simulink model "test_integration_decrease_power"  (R2022b)
settings: Solver=FixedStepAuto  StartTime=0.0  StopTime=240  FixedStep=0.1  RelTol=1e-3
settings Model: Creator=cristian  LastModifiedBy=cristian
settings ConfigComp: CovScope=ReferencedModels  CovIncludeTopModel=off  CovHTMLOptions=-sRT=1 -sVT=0 -aTS=1 -agT=1 -bRG=1 -bTC=1 -hTR=0 -nFC=0 -nFD=1 -scm=1 -bcm=1 -xEv=0 -xEM=0 -req=1  CovEnableCumulative=off

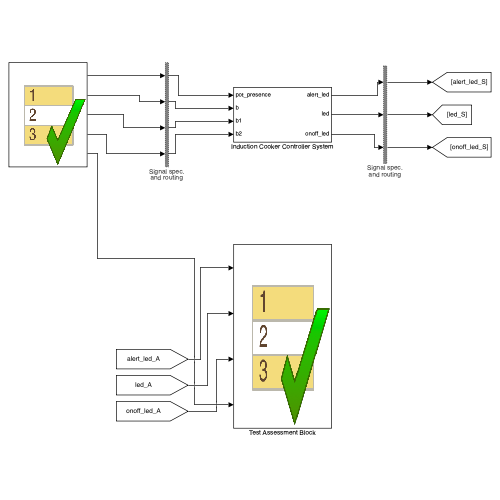
[thumbnail: Simulink's stored preview of the top-level diagram]
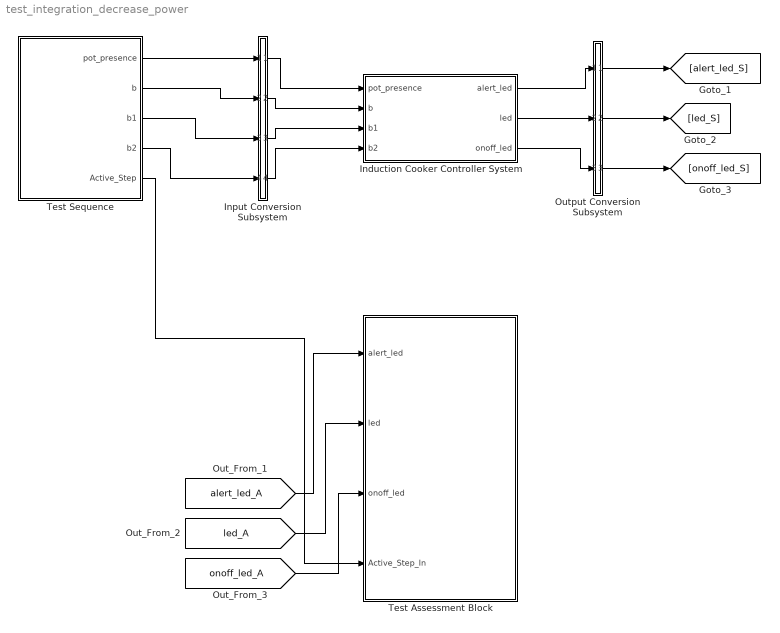
== system test_integration_decrease_power ==
  Induction Cooker Controller System : Subsystem
  Input Conversion Subsystem : Subsystem  Tag=__SLT_ICS__  Description=|
      | Signal spec.
      | and routing
      settings: AttributesFormatString=%<Description>
  Output Conversion Subsystem : Subsystem  Tag=__SLT_OCS__  Description=|
      | Signal spec.
      | and routing
      settings: AttributesFormatString=%<Description>
  Test Assessment Block : Test Sequence  Tag=__SLT_ASMT__  TreatAsAtomicUnit=on
  Test Sequence : Test Sequence  TreatAsAtomicUnit=on
  wires:
  [alert_led_A] -> Test Assessment Block/1(alert_led)
  [led_A] -> Test Assessment Block/2(led)
  [onoff_led_A] -> Test Assessment Block/3(onoff_led)
  Test Sequence/1(pot_presence) -> Input Conversion Subsystem/1(Inport_1)
  Test Sequence/2(b) -> Input Conversion Subsystem/2(Inport_2)
  Test Sequence/3(b1) -> Input Conversion Subsystem/3(Inport_3)
  Test Sequence/4(b2) -> Input Conversion Subsystem/4(Inport_4)
  Output Conversion Subsystem/1(Outport_1) -> [alert_led_S]
  Output Conversion Subsystem/2(Outport_2) -> [led_S]
  Output Conversion Subsystem/3(Outport_3) -> [onoff_led_S]
  Input Conversion Subsystem/1(Outport_1) -> Induction Cooker Controller System/1(pot_presence)
  Input Conversion Subsystem/2(Outport_2) -> Induction Cooker Controller System/2(b)
  Input Conversion Subsystem/3(Outport_3) -> Induction Cooker Controller System/3(b1)
  Input Conversion Subsystem/4(Outport_4) -> Induction Cooker Controller System/4(b2)
  Induction Cooker Controller System/1(alert_led) -> Output Conversion Subsystem/1(Inport_1)
  Induction Cooker Controller System/2(led) -> Output Conversion Subsystem/2(Inport_2)
  Induction Cooker Controller System/3(onoff_led) -> Output Conversion Subsystem/3(Inport_3)
  Test Sequence/5(Active_Step) -> Test Assessment Block/4(Active_Step_In)

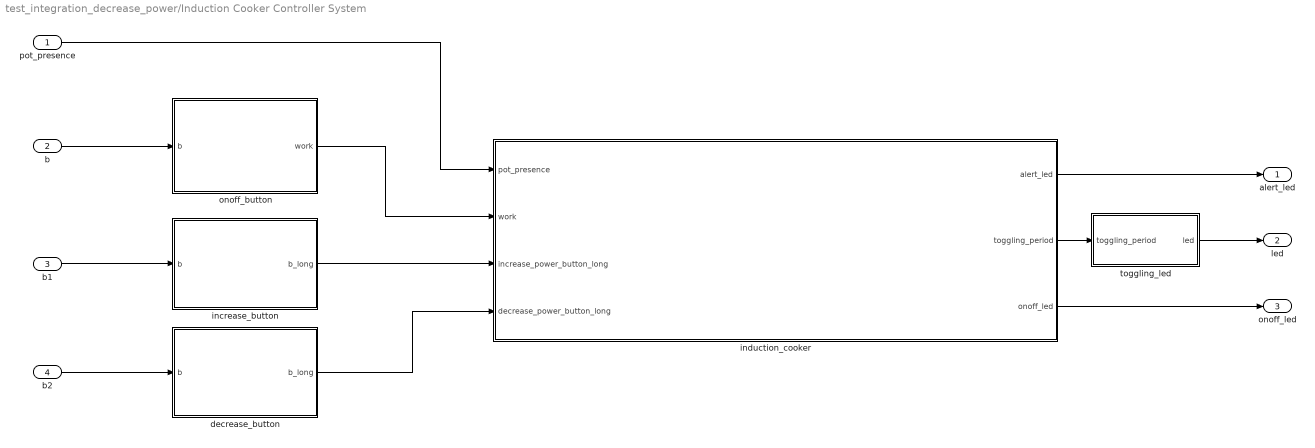
== system test_integration_decrease_power/Induction Cooker Controller System ==
  pot_presence : Inport
  b : Inport  Port=2
  b1 : Inport  Port=3
  b2 : Inport  Port=4
  decrease_button : Stateflow chart  TreatAsAtomicUnit=on
  increase_button : Stateflow chart  TreatAsAtomicUnit=on
  induction_cooker : Stateflow chart  TreatAsAtomicUnit=on
  onoff_button : Stateflow chart  TreatAsAtomicUnit=on
  toggling_led : Stateflow chart  TreatAsAtomicUnit=on
  alert_led : Outport
  led : Outport  Port=2
  onoff_led : Outport  Port=3
  wires:
  decrease_button/1(b_long) -> induction_cooker/4(decrease_power_button_long)
  increase_button/1(b_long) -> induction_cooker/3(increase_power_button_long)
  induction_cooker/2(toggling_period) -> toggling_led/1(toggling_period)
  toggling_led/1(led) -> led/1
  b1/1 -> increase_button/1(b)
  induction_cooker/3(onoff_led) -> onoff_led/1
  onoff_button/1(work) -> induction_cooker/2(work)
  b2/1 -> decrease_button/1(b)
  induction_cooker/1(alert_led) -> alert_led/1
  pot_presence/1 -> induction_cooker/1(pot_presence)
  b/1 -> onoff_button/1(b)

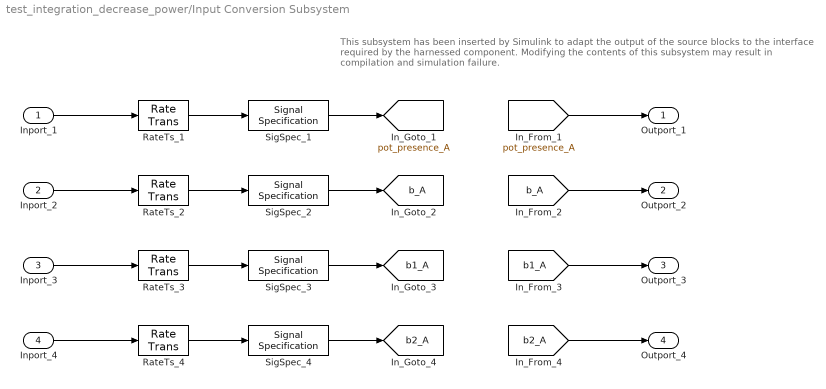
== system test_integration_decrease_power/Input Conversion Subsystem ==
  note: This subsystem has been inserted by Simulink to adapt the output of the source blocks to the interface required by the harnessed component.
      |  Modifying the contents of this subsystem may result in compilation and simulation failure.
  Inport_1 : Inport
  Inport_2 : Inport  Port=2
  Inport_3 : Inport  Port=3
  Inport_4 : Inport  Port=4
  RateTs_{1..4} (4 alike) : RateTransition  OutPortSampleTime=[-1, 0]
  SigSpec_{1..4} (4 alike) : SignalSpecification  OutDataTypeStr=boolean  Dimensions=[1]  SampleTime=[-1, 0]
  Outport_1 : Outport
  Outport_2 : Outport  Port=2
  Outport_3 : Outport  Port=3
  Outport_4 : Outport  Port=4
  tag scope: b1_A=global, b2_A=global, b_A=global, pot_presence_A=global
  wires:
  [pot_presence_A] -> Outport_1/1
  SigSpec_1/1 -> [pot_presence_A]
  RateTs_1/1 -> SigSpec_1/1
  Inport_1/1 -> RateTs_1/1
  [b_A] -> Outport_2/1
  SigSpec_2/1 -> [b_A]
  RateTs_2/1 -> SigSpec_2/1
  Inport_2/1 -> RateTs_2/1
  [b1_A] -> Outport_3/1
  SigSpec_3/1 -> [b1_A]
  RateTs_3/1 -> SigSpec_3/1
  Inport_3/1 -> RateTs_3/1
  [b2_A] -> Outport_4/1
  SigSpec_4/1 -> [b2_A]
  RateTs_4/1 -> SigSpec_4/1
  Inport_4/1 -> RateTs_4/1

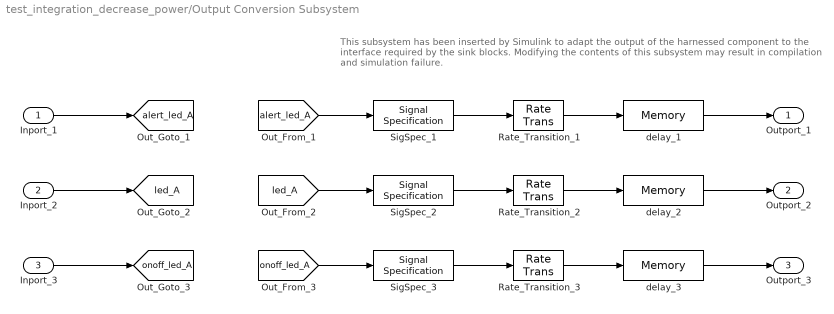
== system test_integration_decrease_power/Output Conversion Subsystem ==
  note: This subsystem has been inserted by Simulink to adapt the output of the harnessed component to the interface required by the sink blocks.
      |  Modifying the contents of this subsystem may result in compilation and simulation failure.
  Inport_1 : Inport
  Inport_2 : Inport  Port=2
  Inport_3 : Inport  Port=3
  Rate_Transition_1 : RateTransition  OutPortSampleTimeOpt=Inherit
  Rate_Transition_2 : RateTransition  OutPortSampleTimeOpt=Inherit
  Rate_Transition_3 : RateTransition  OutPortSampleTimeOpt=Inherit
  SigSpec_1 : SignalSpecification  OutDataTypeStr=boolean  Dimensions=[1]
  SigSpec_2 : SignalSpecification  OutDataTypeStr=boolean  Dimensions=[1]
  SigSpec_3 : SignalSpecification  OutDataTypeStr=boolean  Dimensions=[1]
  delay_1 : Memory
  delay_2 : Memory
  delay_3 : Memory
  Outport_1 : Outport
  Outport_2 : Outport  Port=2
  Outport_3 : Outport  Port=3
  tag scope: alert_led_A=global, led_A=global, onoff_led_A=global
  wires:
  Inport_1/1 -> [alert_led_A]
  [alert_led_A] -> SigSpec_1/1
  SigSpec_1/1 -> Rate_Transition_1/1
  Rate_Transition_1/1 -> delay_1/1
  delay_1/1 -> Outport_1/1
  Inport_2/1 -> [led_A]
  [led_A] -> SigSpec_2/1
  SigSpec_2/1 -> Rate_Transition_2/1
  Rate_Transition_2/1 -> delay_2/1
  delay_2/1 -> Outport_2/1
  Inport_3/1 -> [onoff_led_A]
  [onoff_led_A] -> SigSpec_3/1
  SigSpec_3/1 -> Rate_Transition_3/1
  Rate_Transition_3/1 -> delay_3/1
  delay_3/1 -> Outport_3/1

== stateflow chart test_integration_decrease_power/Induction Cooker Controller System/decrease_button ==
  note: Bottone a livelli, la pressione per un numero di secondi pari a DURATION permette di avere un uscita alta in maniera istantanea.
      | Per avere in output un valore PRESSED, è necessare lasciare il bottone e premere tra un output e l'altro.
  state Wait
    en: b_long = RELEASED
  state Pressed
    en: b_long = RELEASED;
    on after(DURATION,sec): b_long = PRESSED
  state LongPressed
    en: b_long = RELEASED
  (default) -> Wait
  Wait -> Pressed : [b == PRESSED]
  Pressed -> Wait [order 1] : [b == RELEASED]
  LongPressed -> Wait : [b == RELEASED]
  Pressed -> LongPressed [order 2] : [b_long == PRESSED && b == PRESSED]
  data: b_long output boolean size=1; PRESSED constant boolean size=1 =0; RELEASED constant boolean size=1 =1; b input boolean size=1; DURATION constant double size=1 =1

== stateflow chart test_integration_decrease_power/Induction Cooker Controller System/increase_button ==
  note: Bottone a livelli, la pressione per un numero di secondi pari a DURATION permette di avere un uscita alta in maniera istantanea.
      | Per avere in output un valore PRESSED, è necessare lasciare il bottone e premere tra un output e l'altro.
  state Wait
    en: b_long = RELEASED
  state Pressed
    en: b_long = RELEASED;
    on after(DURATION,sec): b_long = PRESSED
  state LongPressed
    en: b_long = RELEASED
  (default) -> Wait
  Wait -> Pressed : [b == PRESSED]
  Pressed -> Wait [order 1] : [b == RELEASED]
  LongPressed -> Wait : [b == RELEASED]
  Pressed -> LongPressed [order 2] : [b_long == PRESSED && b == PRESSED]
  data: b_long output boolean size=1; PRESSED constant boolean size=1 =0; RELEASED constant boolean size=1 =1; b input boolean size=1; DURATION constant double size=1 =1

== stateflow chart test_integration_decrease_power/Test Sequence ==
  settings: updateMethod=DISCRETE  sampleTime=0.1
  state DecreasePower
    state DP_Init
      %% Initialize data outputs.
      pot_presence = true;
      b = true;
      b1 = true;
      b2 = true;
      settings: description=Inizialmente il fornello è spento.
    state DP_TurnON
      pot_presence = true;
      b = false;
      b1 = true;
      b2 = true;
      settings: description=Accendiamo il fornello, premendo l'apposito pulsante di accensione. Il passaggio avveiene in maniera istantanea.
    state DP_IncreasePower300W
      pot_presence = false;
      b = true;
      b1 = false;
      b2 = true;
      settings: description=Posizioniamo la pentola ed accendiamo il fornello facendo pressione per 1 secondo sull'apposito pulsante di aumento potenza.
    state DP_Wait300W
      pot_presence = false;
      b = true;
      b1 = true;
      b2 = true;
      settings: description=Attendiamo 5 sec affinché il cambiamento diventi effettivo.
    state DP_Set300W
      pot_presence = false;
      b = true;
      b1 = true;
      b2 = true;
      settings: description=Il cambiamento di potenza viene effettuato.
    state DP_DecreasePower0W
      pot_presence = false;
      b = true;
      b1 = true;
      b2 = false;
      settings: description=Facciamo pressione per 1 secondo sull'apposito pulsante di diminuzione di potenza.
    state DP_Wait0W
      pot_presence = false;
      b = true;
      b1 = true;
      b2 = true;
      settings: description=Attendiamo 5 sec affinché il cambiamento diventi effettivo.
    state DP_Set0W
      pot_presence = false;
      b = true;
      b1 = true;
      b2 = true;
      settings: description=Il cambiamento di potenza viene effettuato.
    state DP_void
    (default) -> DP_Init
    DP_Init -> DP_TurnON : [
        | true
        | ]
    DP_TurnON -> DP_IncreasePower300W : [
        | true
        | ]
    DP_IncreasePower300W -> DP_Wait300W : [
        | after(1+SamplePeriod,sec)
        | ]
    DP_Wait300W -> DP_Set300W : [
        | after(5-SamplePeriod,sec)
        | ]
    DP_Set300W -> DP_DecreasePower0W : [
        | true
        | ]
    DP_DecreasePower0W -> DP_Wait0W : [
        | after(1+SamplePeriod,sec)
        | ]
    DP_Wait0W -> DP_Set0W : [
        | after(5-SamplePeriod,sec)
        | ]
    DP_Set0W -> DP_void : [
        | true
        | ]
  (default) -> DecreasePower : {assert(Active_Scenario_Index == 1,'The value of Scenario Parameter ''Active_Scenario_Index'' is not valid. Use the index of the scenario to specify it.')}
  data: pot_presence output boolean size=[1]; b output boolean size=[1]; b1 output boolean size=[1]; b2 output boolean size=[1]; Active_Step output Enum: ActiveStepInt; SamplePeriod constant double =str2num(get_param('InductionCooker','FixedStep')); Active_Scenario_Index parameter =1

== stateflow chart test_integration_decrease_power/Induction Cooker Controller System/induction_cooker ==
  note: Il core del fornello è composto da un chart principale che oscilla tra uno stato ON ed uno stato OFF, a seconda dell'input work che ne indica in che stato di funzionamento deve essere (associato al bottone a livelli di on/off).
  state OFF
    en: onoff_led = LOW, alert_led = LOW,
    current_power = 0, toggling_period = TOGGLING_PERIOD_OFF
  note: Lo stato ON è composto da tre macchine parallele che gestiscono rispettivamente: cambiamento potenza, allarme e blink del led.
  state ON
    state LOGIC [parallel]
      settings: executionOrder=1
      note: In LOGIC, lo stato di ingresso è quello a 0W, in quanto appena accendiamo il fornello esso non è attivo.
          | Quando si riceve l'input di INCREASE o DECREASE button, si transita in uno stato che rappresenta una nuova potenza selezionata, dopo 5 secondi da un passaggio di stato la potenza reale diventerà quella associata allo stato correntemente attivo.
          | Quando una certa potenza viene selezionata, viene aggiornato il periodo di blink del power_led.
      state P0W
        state WAIT
        state SET
          en:
          current_power = 0, toggling_period = TOGGLING_PERIOD_0W
        note: Lo stato che rappresenta 0W gode della particolarità di poter fissare la potenza anche senza attendere i 5s, questo è possibile quando da uno stato gerarchicamente superiore o parallelo viene impostato current_power = 0W. Tale circostanza avviene sia all'avvio in cui non vi è necessità di attendere del tempo prima di impostare la potenza a 0W e sia nel momento in cui scatta l'allarme, in cui si disattiva il fornello istantaneamente.
        (default) -> ON.LOGIC.P0W.WAIT
        ON.LOGIC.P0W.WAIT -> ON.LOGIC.P0W.SET : [after(SET_POWER_PATIENCE,sec) || current_power == 0]
      note: Notiamo che in ogni stato di LOGIC, diverso da 0W, vi è una transizione associata al fatto che la variabile alarm assume valore HIGH, che ci riporta automaticamente nello stato 0W e fissa tale potenza come potenza corrente senza attendere i 10 secondi.
      state P1500W
        state WAIT
        state SET
          en:
          current_power = 1500, toggling_period = TOGGLING_PERIOD_1500W
        (default) -> ON.LOGIC.P1500W.WAIT
        ON.LOGIC.P1500W.WAIT -> ON.LOGIC.P1500W.SET : after(SET_POWER_PATIENCE,sec)
      state P300W
        state WAIT
        state SET
          en:
          current_power = 300, toggling_period = TOGGLING_PERIOD_300W
        (default) -> ON.LOGIC.P300W.WAIT
        ON.LOGIC.P300W.WAIT -> ON.LOGIC.P300W.SET : after(SET_POWER_PATIENCE,sec)
      state P1000W
        state WAIT
        state SET
          en:
          current_power = 1000, toggling_period = TOGGLING_PERIOD_1000W
        (default) -> ON.LOGIC.P1000W.WAIT
        ON.LOGIC.P1000W.WAIT -> ON.LOGIC.P1000W.SET : after(SET_POWER_PATIENCE,sec)
      state P500W
        state WAIT
        state SET
          en:
          current_power = 500, toggling_period = TOGGLING_PERIOD_500W
        (default) -> ON.LOGIC.P500W.WAIT
        ON.LOGIC.P500W.WAIT -> ON.LOGIC.P500W.SET : after(SET_POWER_PATIENCE,sec)
      (default) -> P0W
      P1500W -> P0W [order 2] : [alarm == HIGH]
      P0W -> P300W : [increase_power_button_long == PRESSED && pot_presence == PRESSED]
      P300W -> P0W [order 1] : [(alarm == HIGH) || (decrease_power_button_long == PRESSED && pot_presence == PRESSED)]
      P500W -> P0W [order 3] : [alarm == HIGH]
      P1000W -> P0W [order 3] : [alarm == HIGH]
      P500W -> P300W [order 1] : [decrease_power_button_long == PRESSED && pot_presence == PRESSED]
      P300W -> P500W [order 2] : [increase_power_button_long == PRESSED && pot_presence == PRESSED]
      P1500W -> P1000W [order 1] : [decrease_power_button_long == PRESSED && pot_presence == PRESSED]
      P1000W -> P1500W [order 2] : [increase_power_button_long == PRESSED && pot_presence == PRESSED]
      P500W -> P1000W [order 2] : [increase_power_button_long == PRESSED && pot_presence == PRESSED]
      P1000W -> P500W [order 1] : [decrease_power_button_long == PRESSED && pot_presence == PRESSED]
    state ALARM [parallel]
      settings: executionOrder=2
      state ACTIVE
        state QUIET
          en: alarm = LOW, alert_led = LOW
        state ALARM
          en: alert_led = HIGH
          on after(ALARM_PATIENCE,sec): alarm = HIGH; current_power = 0; toggling_period = TOGGLING_PERIOD_0W; alert_led = LOW;
        (default) -> QUIET
        QUIET -> ON.ALARM.ACTIVE.ALARM : [pot_presence == RELEASED]
        ON.ALARM.ACTIVE.ALARM -> QUIET : [pot_presence == PRESSED]
      state INACTIVE
        en:
        alarm = LOW,
        alert_led = LOW
      (default) -> INACTIVE
      INACTIVE -> ACTIVE : [current_power ~= 0]
      ACTIVE -> INACTIVE : [current_power == 0]
    state TOGGLING_LED [parallel] [commented out]
      note: In ogni stato di LOGIC, che rappresenta una specifica potenza, viene impostato un valore di periodo che indica ogni quanto il power_led (led giallo) lampeggia.
          | Infatti, tale macchina semplicemente rimbalza da uno stato all'altro accendendo e spegnendo il led.
      state LED_OFF [commented out]
        en: power_led=LOW;
      state LED_ON [commented out]
        en: power_led=HIGH;
      (default) -> LED_OFF [commented out]
      LED_OFF -> LED_ON [commented out] : [toggling_period>0 && after(toggling_period,sec)]
      LED_ON -> LED_OFF [commented out] : [after(toggling_period,sec)]
  note: Quando la macchina non è attiva (current_power = 0W), anche l'allarme è inattivo. All'attivazione del fornello corrisponde l'attivazione dell'allarme.
      | Nel momento in cui l'allarme è attivo e rileva una rimozione della pentola passa in uno stato ALARM che accende l'alert_led e dopo 10 secondi di permanenza disattiva il sistema portando LOGIC nello stato 0W, a meno di reinserimento pentola che riporta in uno stato QUIET.
  (default) -> OFF
  OFF -> ON : [work == HIGH]{onoff_led = HIGH}
  ON -> OFF : [work == LOW]
  data: pot_presence input boolean size=1; work input boolean size=1; alarm local boolean size=1; alert_led output boolean size=1; toggling_period output double size=1; onoff_led output boolean size=1; current_power local uint16 size=1; increase_power_button_long input boolean size=1; decrease_power_button_long input boolean size=1; HIGH constant boolean size=1 =1; PRESSED constant boolean size=1 =0; RELEASED constant boolean size=1 =1; LOW constant boolean size=1 =0; ALARM_PATIENCE constant double =10; TOGGLING_PERIOD_0W constant double =0; TOGGLING_PERIOD_300W constant double =2; TOGGLING_PERIOD_500W constant double =1; TOGGLING_PERIOD_1000W constant double =0.5; TOGGLING_PERIOD_1500W constant double =0.25; SET_POWER_PATIENCE local =5; TOGGLING_PERIOD_OFF constant double =0

== stateflow chart test_integration_decrease_power/Induction Cooker Controller System/onoff_button ==
  note: Stato di accensione del bottone onoff
  note: In questo stato il bottone può accendere la macchina
  state INACTIVE
    state Pressed
      en: work = HIGH
    state Wait
      en: work = LOW
    (default) -> INACTIVE.Wait
    INACTIVE.Wait -> INACTIVE.Pressed : [b == PRESSED]
  note: Stato di spegnimento del bottone onoff
  note: In questo stato il bottone può spengere la macchina
  state ACTIVE
    state Wait
      en:
      b_long = RELEASED
    state Pressed
      en:
      b_long = RELEASED;
      on after(DURATION,sec): b_long = PRESSED
    state LongPressed
      en: work = LOW;
    (default) -> ACTIVE.Wait
    ACTIVE.Wait -> ACTIVE.Pressed : [b == PRESSED]
    ACTIVE.Pressed -> ACTIVE.Wait [order 1] : [b == RELEASED]
    ACTIVE.Pressed -> LongPressed [order 2] : [b_long == PRESSED && b == PRESSED]
  note: Se il bottone viene premuto una sola volta, il sistema viene acceso.
      | Se il bottone viene premuto per 1 secondo, il sistema viene spento.
      | Una pressione prolungata senza rilascio del bottone, non causa un alternarsi di accensioni e spegnimenti continui.
  (default) -> INACTIVE
  INACTIVE.Pressed -> ACTIVE : [b == RELEASED]
  LongPressed -> INACTIVE : [b==RELEASED]
  data: PRESSED constant boolean size=1 =0; RELEASED constant boolean size=1 =1; b input boolean size=1; DURATION constant double size=1 =1; b_long local boolean size=1; HIGH constant boolean size=1 =1; LOW constant boolean size=1 =0; work output boolean size=1

== stateflow chart test_integration_decrease_power/Induction Cooker Controller System/toggling_led ==
  note: Lo spegnimento ha invece la priorità, appena ho periodo=0 spengo.
  state Off
    en: led = LOW
  state Blink_Off
    en:
    led = LOW
    period = toggling_period
  state Blink_On
    en:
    led = HIGH
    period = toggling_period
  note: L'utilizzo di una variabile di appoggio consente di gestire il caso in cui durante il blinking il periodo viene cambiato. Usando tale variabile, lo stato corrente viene termianto dopo un'attesa pari al vecchio periodo e dal nuovo stato vi sarà la variazione di periodo.
      | Ad esempio, se passo da 1s a 2s, ed attualmente il led è acceso, lo spegnerò terminando l'attesa di 1s e dal prossimo stato l'attesa sarà di 2s.
  (default) -> Off
  Blink_Off -> Off [order 1] : [toggling_period == 0]
  Blink_On -> Off [order 1] : [toggling_period == 0]
  Off -> Blink_On : [toggling_period ~= 0]
  Blink_On -> Blink_Off [order 2] : [after(period,sec)]
  Blink_Off -> Blink_On [order 2] : [after(period,sec)]
  data: toggling_period input double; led output boolean; HIGH constant boolean =1; LOW constant boolean =0; period local

== stateflow chart test_integration_decrease_power/Test Assessment Block ==
  state DecreasePower
    state Init
      state Verify_DP_Init
        verify(alert_led==0 && led==0 && onoff_led==0);
        settings: description=|
            | Inizializzazione.
            | Tutti i led sono spenti.
      state Verify_DP_TurnON
        verify(alert_led==0 && led==0 && onoff_led==1);
        settings: description=|
            | Accensione del dispositivo.
            | Il led di accensione è acceso.
      state Verify_DP_IncreasePower300W
        verify(alert_led==0 && led==0 && onoff_led==1);
        settings: description=|
            | Richiesta di aumento della potenza.
            | Il led di accensione è acceso.
      state Verify_DP_Wait300W
        verify(alert_led==0 && led==0 && onoff_led==1);
        settings: description=|
            | Attesa del cambiamento di potenza.
            | Il led di accensione è acceso.
      state Verify_DP_Set300W
        verify(alert_led==0 && led==1 && onoff_led==1)
        settings: description=|
            | Conferma della nuova potenza.
            | Il led di accensione è acceso ed il led giallo di attivazione sta blinkando con periodo di 2 s.
      state Verify_DP_DecreasePower0W
        verify(alert_led==0 && led==1 && onoff_led==1);
        settings: description=|
            | Richiesta di decremento della potenza.
            | Il led di accensione è acceso ed il led giallo di attivazione sta blinkando con periodo di 2 s.
      state Verify_DP_Wait0W
        settings: description=Attesa del cambiamento di potenza.
        state Verify__DP_Wait0W_1
          verify(alert_led==0 && led==1 && onoff_led==1);
          settings: description=led giallo di attivazione on
        state Verify_DP_Wait0W_2
          verify(alert_led==0 && led==0 && onoff_led==1);
          settings: description=led giallo di attivazione off
        state Verify_DP_Wait0W_3
          verify(alert_led==0 && led==1 && onoff_led==1);
          settings: description=led giallo di attivazione on
        state Verify_DP_Wait0W_4
          verify(alert_led==0 && led==0 && onoff_led==1);
          settings: description=led giallo di attivazione off
        (default) -> Verify__DP_Wait0W_1
        Verify__DP_Wait0W_1 -> Verify_DP_Wait0W_2 : [
            | after(2-(1+2*SamplePeriod),sec)
            | ]
        Verify_DP_Wait0W_2 -> Verify_DP_Wait0W_3 : [
            | after(2,sec)
            | ]
        Verify_DP_Wait0W_3 -> Verify_DP_Wait0W_4 : [
            | after(2,sec)
            | ]
      state Verify_DP_Set0W
        verify(alert_led==0 && led==0 && onoff_led==1)
        settings: description=|
            | Conferma della nuova potenza di 0W.
            | Il led giallo di attivazione torna ad essere spento, mentre il verde di accensione è acceso.
      state Init_1
      Init -> (junction 349)
      (default) -> (junction 349)
      (junction 349) -> (junction 350) [order 1] : [Active_Step_In == ActiveStepInt.DP_Init
          | ]
      (junction 350) -> Verify_DP_Init [order 1] : [~in(DecreasePower.Init.Verify_DP_Init)]
      (junction 349) -> (junction 359) [order 2]
      (junction 350) -> (junction 353) [order 2]
      (junction 359) -> (junction 360) [order 1] : [Active_Step_In == ActiveStepInt.DP_TurnON
          | ]
      (junction 360) -> Verify_DP_TurnON [order 1] : [~in(DecreasePower.Init.Verify_DP_TurnON)]
      (junction 359) -> (junction 367) [order 2]
      (junction 360) -> (junction 363) [order 2]
      (junction 367) -> (junction 368) [order 1] : [Active_Step_In == ActiveStepInt.DP_IncreasePower300W
          | ]
      (junction 368) -> Verify_DP_IncreasePower300W [order 1] : [~in(DecreasePower.Init.Verify_DP_IncreasePower300W)]
      (junction 367) -> (junction 375) [order 2]
      (junction 368) -> (junction 371) [order 2]
      (junction 375) -> (junction 376) [order 1] : [Active_Step_In == ActiveStepInt.DP_Wait300W
          | ]
      (junction 376) -> Verify_DP_Wait300W [order 1] : [~in(DecreasePower.Init.Verify_DP_Wait300W)]
      (junction 375) -> (junction 383) [order 2]
      (junction 376) -> (junction 379) [order 2]
      (junction 383) -> (junction 384) [order 1] : [Active_Step_In == ActiveStepInt.DP_Set300W
          | ]
      (junction 384) -> Verify_DP_Set300W [order 1] : [~in(DecreasePower.Init.Verify_DP_Set300W)]
      (junction 383) -> (junction 391) [order 2]
      (junction 384) -> (junction 387) [order 2]
      (junction 391) -> (junction 392) [order 1] : [Active_Step_In == ActiveStepInt.DP_DecreasePower0W
          | ]
      (junction 392) -> Verify_DP_DecreasePower0W [order 1] : [~in(DecreasePower.Init.Verify_DP_DecreasePower0W)]
      (junction 391) -> (junction 399) [order 2]
      (junction 392) -> (junction 395) [order 2]
      (junction 399) -> (junction 400) [order 1] : [Active_Step_In == ActiveStepInt.DP_Wait0W
          | ]
      (junction 400) -> Verify_DP_Wait0W [order 1] : [~in(DecreasePower.Init.Verify_DP_Wait0W)]
      (junction 399) -> (junction 416) [order 2]
      (junction 400) -> (junction 403) [order 2]
      (junction 416) -> (junction 417) [order 1] : [Active_Step_In == ActiveStepInt.DP_Set0W
          | ]
      (junction 417) -> Verify_DP_Set0W [order 1] : [~in(DecreasePower.Init.Verify_DP_Set0W)]
      (junction 417) -> (junction 420) [order 2]
      (junction 424) -> (junction 425)
      (junction 425) -> Init_1 [order 1] : [~in(DecreasePower.Init.Init_1)]
      (junction 425) -> (junction 428) [order 2]
      (junction 416) -> (junction 424) [order 2]
    (default) -> Init
  (default) -> DecreasePower : {assert(Active_Scenario_Index == 1,'The value of Scenario Parameter ''Active_Scenario_Index'' is not valid. Use the index of the scenario to specify it.')}
  data: alert_led input boolean size=[1]; led input boolean size=[1]; onoff_led input boolean size=[1]; Active_Step_In input; Active_Scenario_Index parameter =1; SamplePeriod constant double =str2num(get_param('InductionCooker','FixedStep'))
